simulink model "PowE_lab4_1_fullwaveSInglephaseuncRectifier"  (R2021b)
settings: Solver=VariableStepAuto  StartTime=0.0  StopTime=0.5  RelTol=1e-3
libraries: spsDiodeLib x4, spsVoltageMeasurementLib x3, spsACVoltageSourceLib x1, spsCurrentMeasurementLib x1, spsDCVoltageSourceLib x1, spsMeanLib x1, spsRMSLib x1, spsSeriesRLCBranchLib x1, spspowerguiLib x1
settings Model: Creator=kumaraditya  LastModifiedBy=Asus

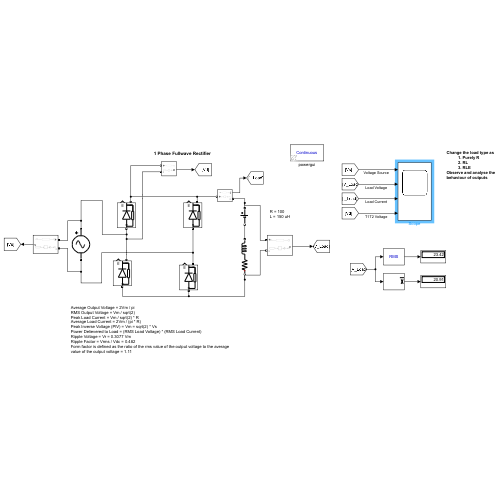
[thumbnail: Simulink's stored preview of the top-level diagram]
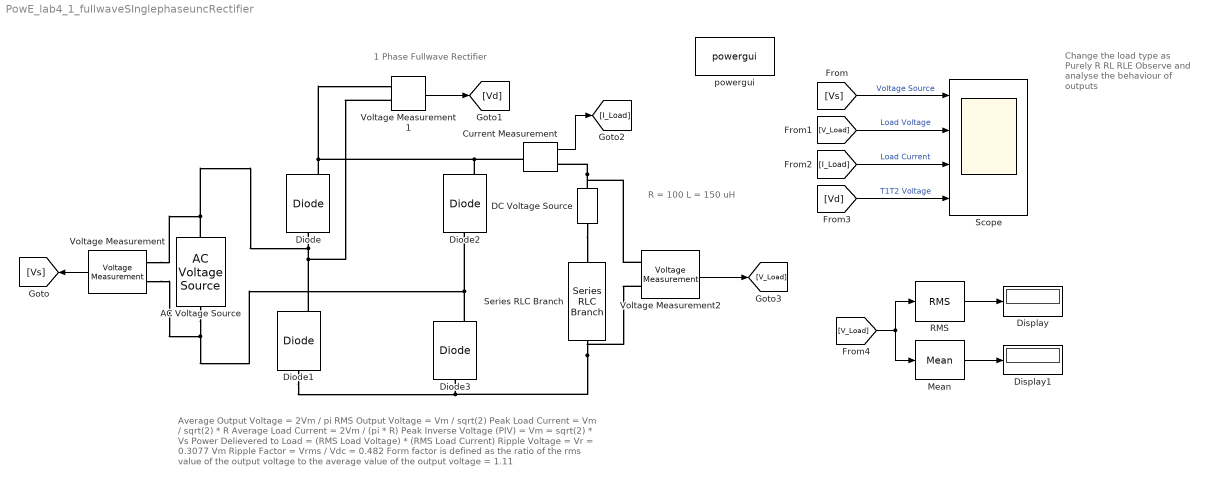
== system PowE_lab4_1_fullwaveSInglephaseuncRectifier ==
  note: 1 Phase Fullwave Rectifier
  note: Average Output Voltage = 2Vm / pi
      | RMS Output Voltage = Vm / sqrt(2)
      | Peak Load Current = Vm / sqrt(2) * R
      | Average Load Current = 2Vm / (pi * R)
      | Peak Inverse Voltage (PIV) = Vm = sqrt(2) * Vs
      | Power Delievered to Load = (RMS Load Voltage) * (RMS Load Current)
      | Ripple Voltage = Vr = 0.3077 Vm
      | Ripple Factor = Vrms / Vdc = 0.482
      | Form factor is defined as the ratio of the rms value of the output voltage to the average value of the output voltage = 1.11
  note: R = 100
      | L = 150 uH
  note: Change the load type as
      | Purely R
      | RL
      | RLE
      | Observe and analyse the
      | behaviour of outputs
  AC Voltage Source : spsACVoltageSourceLib/AC Voltage Source  Amplitude=34  Phase=0  Frequency=50  SampleTime=0  Measurements=None  BusType=swing  Pref=10e3  Qref=0  Qmin=-inf  Qmax=+inf
  Current Measurement : spsCurrentMeasurementLib/Current Measurement  PhasorSimulation=off  OutputType=Complex  PSBequivalent=0
  DC Voltage Source : spsDCVoltageSourceLib/DC Voltage Source  Amplitude=0  Measurements=Voltage
  Diode{,1..3} (4 alike) : spsDiodeLib/Diode  Ron=0.001  Lon=0  Vf=0.8  IC=0  UseSnubber=0  Rs=500  Cs=250e-9  Measurements=on
  Display : Display
  Display1 : Display
  Mean : spsMeanLib/Mean  Freq=60  Vinit=0  Ts=0
  RMS : spsRMSLib/RMS  TrueRMS=on  Freq=60  RMSInit=120  Ts=0
  Scope : Scope  NumInputPorts=4
  Series RLC Branch : spsSeriesRLCBranchLib/Series RLC Branch  LConnTagsString=__new0  RConnTagsString=__new0  BranchType=RL  Resistance=100  Inductance=150e-6  SetiL0=off  InitialCurrent=0  Capacitance=1e-6  Setx0=off  InitialVoltage=0  Measurements=None
  Voltage Measurement : spsVoltageMeasurementLib/Voltage Measurement  PhasorSimulation=off  OutputType=Complex  PSBequivalent=0
  Voltage Measurement1 : spsVoltageMeasurementLib/Voltage Measurement  PhasorSimulation=off  OutputType=Complex  PSBequivalent=0
  Voltage Measurement2 : spsVoltageMeasurementLib/Voltage Measurement  PhasorSimulation=off  OutputType=Complex  PSBequivalent=0
  powergui : spspowerguiLib/powergui  Priority=1  SimulationMode=Continuous  SampleTime=50e-6  frequency=60  Iterations=50  frequencyindice=50  Pbase=100e6  ErrMax=1e-4  UnitsV=kV  UnitsW=MW  buscounter=0  FunctionMessages=off  echomessages=off  EnableUseOfTLC=off  CurrentSourceSwitches=off  DisableSnubberDevices=off  DisableRonSwitches=off  DisableVfSwitches=off  DisplayEquations=off  AutomaticDiscreteSolvers=off  SolverType=Tustin/Backward Euler (TBE)  Interpol=off  ExternalGateDelay=off  methode=off  Ts=100  x0status=blocks  SPID=on  SwTol=0  HookPort=off  NonlinearTolerance=1e-4  nMaxIteration=100  ContinueOnMaxIteration=off  RestoreLinks=warning  ResistiveCurrentMeasurement=off  Frange=[0:2:500]  Ylog=off  Xlog=on  ShowGrid=off  save=off  variable=ZData  structure=0  ZoomFFT=off  StartTime=0.0  cycles=1  DisplayStyle=1  fundamental=60  FreqAxis=off  MaxFrequency=1000  frequencyindicesteady=1  RmsSteady=1  display=off
  wires:
  Voltage Measurement/1 -> [Vs]
  Voltage Measurement1/1 -> [Vd]
  Current Measurement/1 -> [I_Load]
  Voltage Measurement2/1 -> [V_Load]
  [Vs] -> Scope/1  "Voltage Source"
  [V_Load] -> Scope/2  "Load Voltage"
  [I_Load] -> Scope/3  "Load Current"
  [Vd] -> Scope/4  "T1T2 Voltage"
  [V_Load] -> RMS/1, Mean/1
  RMS/1 -> Display/1
  Mean/1 -> Display1/1
  connections:
  Diode1/RConn1 -- Voltage Measurement1/LConn2 -- Voltage Measurement/LConn1 -- AC Voltage Source/RConn1 -- Diode/LConn1
  Diode3/RConn1 -- Voltage Measurement/LConn2 -- AC Voltage Source/LConn1 -- Diode2/LConn1
  Diode/RConn1 -- Current Measurement/LConn1 -- Diode2/RConn1 -- Voltage Measurement1/LConn1
  Series RLC Branch/LConn1 -- Voltage Measurement2/LConn2 -- Diode1/LConn1 -- Diode3/LConn1
  DC Voltage Source/RConn1 -- Current Measurement/RConn1 -- Voltage Measurement2/LConn1
  DC Voltage Source/LConn1 -- Series RLC Branch/RConn1
